simulink model "CM690A_HwAg0Meas"  (R2013b)
settings: Solver=FixedStepDiscrete  SolverMode=SingleTasking  StartTime=0.0  StopTime=22  FixedStep=0.002  RelTol=1e-3
undefined symbols (not defined in the file): ELECGLBPRM_DEGPERREV_DEGPERREV_F32, ELECGLBPRM_HWAGCENTROFFS_HWDEG_F32, ELECGLBPRM_HWAGSATNLOWRLIM_HWDEG_F32, ELECGLBPRM_HWAGSATNUPPRLIM_HWDEG_F32, ELECGLBPRM_HWAGSCA_ULS_F32, ELECGLBPRM_HWAGSPURGEARRAT_ULS_F32, ELECGLBPRM_HWAGSPURTORINGGEARRATSNSR0_ULS_F32, ELECGLBPRM_HWAGSPURTORINGGEARRATSNSR1_ULS_F32, ELECGLBPRM_NOFLT_CNT_U08, ELECGLBPRM_OFFSTRIMNOTPRFMD_CNT_U08, ELECGLBPRM_PRTCLFLT_CNT_U08, ELECGLBPRM_SKIPSTEPFLT_CNT_U08, ELECGLBPRM_SNSRINTFLT_CNT_U08, ELECGLBPRM_VRNRERRFLT_CNT_U08, FLTINJ_HWAG0MEAS_HWAG0, FLTINJ_HWAG0MEAS_TESTOK, HwAg0IfFlt, HwAg0MeasHwAg0IfFltFailStep, HwAg0MeasHwAg0IfFltPassStep, HwAg0MeasHwAg0Snsr0PrtclFltFailStep, HwAg0MeasHwAg0Snsr0PrtclFltPassStep, HwAg0MeasHwAg0Snsr1PrtclFltFailStep, HwAg0MeasHwAg0Snsr1PrtclFltPassStep, HwAg0MeasSnsr0Rev, HwAg0MeasSnsr1Rev, HwAg0MeasStep, HwAg0MeasVrnrErrThd, HwAg0MfgFlt, HwAg0Snsr0PrtclFlt, HwAg0Snsr1PrtclFlt, HWAG10THTOOTHTRIG_CNT_U08, HWAG11THTOOTHTRIG_CNT_U08, NtcSts1, sigbuilder_block, SigQlfr1
libraries: simulink x30, NxtrNvM x3
(part 4 of 5)

== system CM690A_HwAg0Meas/HwAg0Meas/HwAg0MeasPer2/Snsr0Read/RawHwAgRead/CopyRight2 ==

== system CM690A_HwAg0Meas/HwAg0Meas/HwAg0MeasPer2/Snsr0Read/RawHwAgRead/NewMsg ==
  note: Information Only:
      |
      | - Protocol Fault Evaluation
  note: ,
  note: Fault
      | Injection
      | Point
  Snsr0CS : Inport
  Snsr0FCCN : Inport  Port=2
  Snsr0Id : Inport  Port=3
  Snsr0Data : Inport  Port=4
  Action Port : ActionPort  ActionType=then
  Bus Creator : BusCreator  Inputs=3
  Bus Selector : BusSelector  OutputSignals=RawHwAg,TestOk,ParamByte
  Bus Selector1 : BusSelector  OutputSignals=RawHwAg,TestOk,ParamByte
  CopyRight2 : Subsystem  Description=|  mask(Copyright Information){none=on}
      | Copyright info block.                                               
      |                                                                     
      | Place copyright information at the top of every subsystem in design.
      mask prompts: none "No parameters"
      mask help: Place copyright information at the top of every subsystem in design.
      mask Display:
      | NxtrConf = 'Nexteer Confidential';
      | 
      | sys = bdroot; %handle for the current model ("system")
      | first = get_param(sys,'Created');
      | first = first(end-3:end);  %year is last four digits
      | 
      | last = get_param(sys,'LastModifiedDate');
      | if isempty(last)
      |     last = datestr(now,'yyyy');
      | else
      |     last = last(end-3:end);
      | end
      | 
      | if strcmp(first,last)
      |     fprintf('%s -- Copyright %s Nexteer',NxtrConf,first)
      | else
      |     fprintf('%s -- %s%s- %s Nexteer',NxtrConf,char(169),first,last)
      | end
  FIU : Constant  Value=FLTINJ_HWAG0MEAS_TESTOK
  FltInj_u08 : Subsystem  RequirementInfo={'linktype_rmi_doors' '0000cf45 (/ESG Group/FDD Module Requirements/EA4 Specific/CM690A_HwAg0Meas)' '#CM690A_109' 'true' 'REQ: CM690A_109' '' } %GIDa_7b346184_324c_480b_97a4_826e0f4ed5b6  TreatAsAtomicUnit=on  VariantControl=FltInj_sim  mask(Fault_Injection){}
      mask help: Fault Injection is a simulation only block for EA4 programs.
  If : If  RequirementInfo={} %GIDa_02db3ab5_be9b_4d14_aa60_e7f5bf325249  IfExpression=u1 == 0
  Merge : Merge
  Merge1 : Merge
  Merge2 : Merge
  NoStsFlt : Subsystem  RequirementInfo={} %GIDa_b7e9d759_3768_4543_969e_0ff60280fe32  TreatAsAtomicUnit=on
  STSFLT : Subsystem  RequirementInfo={'linktype_rmi_doors' '0000cf45 (/ESG Group/FDD Module Requirements/EA4 Specific/CM690A_HwAg0Meas)' '#CM690A_40' 'true' 'REQ: CM690A_40' '' ; 'linktype_rmi_doors' '0000cf45 (/ESG Group/FDD Module Requirements/EA4 Specific/CM690A_HwAg0Meas)' '#CM690A_41' 'true' 'REQ: CM690A_41' '' ; 'linktype_rmi_doors' '0000cf45 (/ESG Group/FDD Module Requirements/EA4 Specific/CM690A_HwAg0Meas)' '#CM690A_42' 'true' 'REQ: CM690A_42' '' ; 'linktype_rmi_doors' '0000cf45 (/ESG Group/FDD Module Requirements/EA4 Specific/CM690A_HwAg0Meas)' '#CM690A_43' 'true' 'REQ: CM690A_43' '' ; 'linktype_rmi_doors' '0000cf45 (/ESG Group/FDD Module Requirements/EA4 Specific/CM690A_HwAg0Meas)' '#CM690A_44' 'true' 'REQ: CM690A_44' '' ; 'linktype_rmi_doors' '0000cf45 (/ESG Group/FDD Module Requirements/EA4 Specific/CM690A_HwAg0Meas)' '#CM690A_89' 'true' 'REQ: CM690A_89' '' ; 'linktype_rmi_doors' '0000cf45 (/ESG Group/FDD Module Requirements/EA4 Specific/CM690A_HwAg0Meas)' '#CM690A_45' 'true' 'REQ: CM690A_45' '' ; 'linktype_rmi_doors' '0000cf45 (/ESG Group/FDD Module Requirements/EA4 Specific/CM690A_HwAg0Meas)' '#CM690A_46' 'true' 'REQ: CM690A_46' '' } %GIDa_15585e29_68a1_46d0_9954_0916d9066e3c  TreatAsAtomicUnit=on
      mask Display: disp('STSFLT')
  Out1 : Outport
  wires:
  Snsr0CS/1 -> FltInj_u08/1(Signal)
  If/1 -> NoStsFlt/Action  "NoFault"
  If/2 -> STSFLT/Action  "Fault"
  Merge/1 -> Bus Creator/2  "TestOk"
  Merge1/1 -> Bus Creator/3  "ParamByte"
  Merge2/1 -> Bus Creator/1  "RawHwAg"
  NoStsFlt/1(Out1) -> Bus Selector/1
  STSFLT/1(Out1) -> Bus Selector1/1
  Bus Selector1/1 -> Merge2/1  "<RawHwAg>"
  Bus Selector/1 -> Merge2/2  "<RawHwAg>"
  Bus Selector1/2 -> Merge/1  "<TestOk>"
  Bus Selector1/3 -> Merge1/1  "<ParamByte>"
  Bus Selector/2 -> Merge/2  "<TestOk>"
  Bus Selector/3 -> Merge1/2  "<ParamByte>"
  Bus Creator/1 -> Out1/1
  FIU/1 -> FltInj_u08/2(Const)
  FltInj_u08/1(Out1) -> If/1
  Snsr0FCCN/1 -> NoStsFlt/1(Snsr0FCCN)
  Snsr0Data/1 -> NoStsFlt/3(Snsr0Data)
  Snsr0Id/1 -> NoStsFlt/2(Snsr0Id)

== system CM690A_HwAg0Meas/HwAg0Meas/HwAg0MeasPer2/Snsr0Read/RawHwAgRead/NoNewMsg ==
  Action Port : ActionPort  ActionType=else
  Add : Sum
  Bus Creator : BusCreator  Inputs=3
  Constant : Constant  OutDataTypeStr=uint8
  CopyRight2 : Subsystem  Description=|  mask(Copyright Information){none=on}
      | Copyright info block.                                               
      |                                                                     
      | Place copyright information at the top of every subsystem in design.
      mask prompts: none "No parameters"
      mask help: Place copyright information at the top of every subsystem in design.
      mask Display:
      | NxtrConf = 'Nexteer Confidential';
      | 
      | sys = bdroot; %handle for the current model ("system")
      | first = get_param(sys,'Created');
      | first = first(end-3:end);  %year is last four digits
      | 
      | last = get_param(sys,'LastModifiedDate');
      | if isempty(last)
      |     last = datestr(now,'yyyy');
      | else
      |     last = last(end-3:end);
      | end
      | 
      | if strcmp(first,last)
      |     fprintf('%s -- Copyright %s Nexteer',NxtrConf,first)
      | else
      |     fprintf('%s -- %s%s- %s Nexteer',NxtrConf,char(169),first,last)
      | end
  Data Store Read : DataStoreRead  DataStoreName=HwAg0Snsr0NoMsgErrCntr
  Data Store Write : DataStoreWrite  DataStoreName=HwAg0Snsr0NoMsgErrCntr
  Data Type Conversion : DataTypeConversion  OutDataTypeStr=uint8
  HwAg : Constant  Value=0  OutDataTypeStr=uint16
  NtcSts : simulink/Sources/Enumerated Constant  OutDataTypeStr=Enum: NtcSts1  Value=NtcSts1.NTCSTS_PREFAILD  SampleTime=inf
  PRTCL_FAULT : Constant  Value=ELECGLBPRM_PRTCLFLT_CNT_U08  OutDataTypeStr=uint8
  Signal Conversion : SignalConversion
  Out1 : Outport
  wires:
  PRTCL_FAULT/1 -> Bus Creator/3  "ParamByte"
  NtcSts/1 -> Data Type Conversion/1
  HwAg/1 -> Bus Creator/1  "RawHwAg"
  Bus Creator/1 -> Signal Conversion/1
  Signal Conversion/1 -> Out1/1
  Data Type Conversion/1 -> Bus Creator/2  "TestOk"
  Data Store Read/1 -> Add/1
  Constant/1 -> Add/2
  Add/1 -> Data Store Write/1

== system CM690A_HwAg0Meas/HwAg0Meas/HwAg0MeasPer2/Snsr0Read/Read the Flag/CopyRight2 ==

== system CM690A_HwAg0Meas/HwAg0Meas/HwAg0MeasPer2/Snsr0Read/SetNtcSts/CopyRight2 ==

== system CM690A_HwAg0Meas/HwAg0Meas/HwAg0MeasPer3/Snsr1Read/DebStepSelection/CopyRight2 ==

== system CM690A_HwAg0Meas/HwAg0Meas/HwAg0MeasPer3/Snsr1Read/Do nothing1/CopyRight2 ==

== system CM690A_HwAg0Meas/HwAg0Meas/HwAg0MeasPer3/Snsr1Read/Do nothing2/CopyRight2 ==

== system CM690A_HwAg0Meas/HwAg0Meas/HwAg0MeasPer3/Snsr1Read/RawHwAgRead/CopyRight2 ==

== system CM690A_HwAg0Meas/HwAg0Meas/HwAg0MeasPer3/Snsr1Read/RawHwAgRead/NewMsg ==
  note: Information Only:
      |
      | - Protocol Fault Evaluation
  Snsr1CS : Inport
  Snsr1FCCN : Inport  Port=2
  Snsr1Id : Inport  Port=3
  Snsr1Data : Inport  Port=4
  Action Port : ActionPort  ActionType=then
  Bus Creator : BusCreator  Inputs=3
  Bus Selector : BusSelector  OutputSignals=RawHwAg,TestOk,ParamByte
  Bus Selector1 : BusSelector  OutputSignals=RawHwAg,TestOk,ParamByte
  CopyRight2 : Subsystem  Description=|  mask(Copyright Information){none=on}
      | Copyright info block.                                               
      |                                                                     
      | Place copyright information at the top of every subsystem in design.
      mask prompts: none "No parameters"
      mask help: Place copyright information at the top of every subsystem in design.
      mask Display:
      | NxtrConf = 'Nexteer Confidential';
      | 
      | sys = bdroot; %handle for the current model ("system")
      | first = get_param(sys,'Created');
      | first = first(end-3:end);  %year is last four digits
      | 
      | last = get_param(sys,'LastModifiedDate');
      | if isempty(last)
      |     last = datestr(now,'yyyy');
      | else
      |     last = last(end-3:end);
      | end
      | 
      | if strcmp(first,last)
      |     fprintf('%s -- Copyright %s Nexteer',NxtrConf,first)
      | else
      |     fprintf('%s -- %s%s- %s Nexteer',NxtrConf,char(169),first,last)
      | end
  If : If  RequirementInfo={} %GIDa_d01d7976_4a86_48f6_8a8d_571e55869e77  IfExpression=u1 == 0
  Merge : Merge
  Merge1 : Merge
  Merge2 : Merge
  NoStsFlt : Subsystem  RequirementInfo={} %GIDa_74b744eb_a548_4ce6_ac8b_09cb9d78172d  TreatAsAtomicUnit=on
  STSFLT : Subsystem  RequirementInfo={'linktype_rmi_doors' '0000cf45 (/ESG Group/FDD Module Requirements/EA4 Specific/CM690A_HwAg0Meas)' '#CM690A_57' 'true' 'REQ: CM690A_57' '' ; 'linktype_rmi_doors' '0000cf45 (/ESG Group/FDD Module Requirements/EA4 Specific/CM690A_HwAg0Meas)' '#CM690A_58' 'true' 'REQ: CM690A_58' '' ; 'linktype_rmi_doors' '0000cf45 (/ESG Group/FDD Module Requirements/EA4 Specific/CM690A_HwAg0Meas)' '#CM690A_59' 'true' 'REQ: CM690A_59' '' ; 'linktype_rmi_doors' '0000cf45 (/ESG Group/FDD Module Requirements/EA4 Specific/CM690A_HwAg0Meas)' '#CM690A_60' 'true' 'REQ: CM690A_60' '' ; 'linktype_rmi_doors' '0000cf45 (/ESG Group/FDD Module Requirements/EA4 Specific/CM690A_HwAg0Meas)' '#CM690A_61' 'true' 'REQ: CM690A_61' '' ; 'linktype_rmi_doors' '0000cf45 (/ESG Group/FDD Module Requirements/EA4 Specific/CM690A_HwAg0Meas)' '#CM690A_88' 'true' 'REQ: CM690A_88' '' ; 'linktype_rmi_doors' '0000cf45 (/ESG Group/FDD Module Requirements/EA4 Specific/CM690A_HwAg0Meas)' '#CM690A_62' 'true' 'REQ: CM690A_62' '' ; 'linktype_rmi_doors' '0000cf45 (/ESG Group/FDD Module Requirements/EA4 Specific/CM690A_HwAg0Meas)' '#CM690A_63' 'true' 'REQ: CM690A_63' '' } %GIDa_c06f9169_73b8_4668_a7a1_c8699a32a709  TreatAsAtomicUnit=on
      mask Display: disp('STSFLT')
  Out1 : Outport
  wires:
  If/1 -> NoStsFlt/Action  "NoFault"
  If/2 -> STSFLT/Action  "Fault"
  Merge/1 -> Bus Creator/2  "TestOk"
  Merge1/1 -> Bus Creator/3  "ParamByte"
  Merge2/1 -> Bus Creator/1  "RawHwAg"
  NoStsFlt/1(Out1) -> Bus Selector/1
  STSFLT/1(Out1) -> Bus Selector1/1
  Bus Selector1/1 -> Merge2/1  "<RawHwAg>"
  Bus Selector/1 -> Merge2/2  "<RawHwAg>"
  Bus Selector1/2 -> Merge/1  "<TestOk>"
  Bus Selector1/3 -> Merge1/1  "<ParamByte>"
  Bus Selector/2 -> Merge/2  "<TestOk>"
  Bus Selector/3 -> Merge1/2  "<ParamByte>"
  Bus Creator/1 -> Out1/1
  Snsr1CS/1 -> If/1
  Snsr1FCCN/1 -> NoStsFlt/1(Snsr1FCCN)
  Snsr1Data/1 -> NoStsFlt/3(Snsr1Data)
  Snsr1Id/1 -> NoStsFlt/2(Snsr1Id)

== stateflow chart CM690A_HwAg0Meas/HwAg0Meas/HwAg0MeasPer4/HwAgRead/HwAg0Final/ModRoll ==
  settings: stateMachineType=MEALY_MACHINE
  note: Nexteer Automotive Confidential
  (default) -> (junction 89)
  (junction 89) -> (junction 93) [order 2] : [ RawVal>900 ]
      | {OutVal = RawVal-1800;}
  (junction 89) -> (junction 93) [order 3] : {OutVal = RawVal;}
  (junction 89) -> (junction 93) [order 1] : [RawVal<-900 ]
      | {OutVal = RawVal+1800;}
  data: OutVal output single; RawVal input single

== system CM690A_HwAg0Meas/HwAg0Meas/HwAg0MeasPer3/Snsr1Read/RawHwAgRead/NoNewMsg ==
  Action Port : ActionPort  ActionType=else
  Add : Sum
  Bus Creator : BusCreator  Inputs=3
  Constant : Constant  OutDataTypeStr=uint8
  CopyRight2 : Subsystem  Description=|  mask(Copyright Information){none=on}
      | Copyright info block.                                               
      |                                                                     
      | Place copyright information at the top of every subsystem in design.
      mask prompts: none "No parameters"
      mask help: Place copyright information at the top of every subsystem in design.
      mask Display:
      | NxtrConf = 'Nexteer Confidential';
      | 
      | sys = bdroot; %handle for the current model ("system")
      | first = get_param(sys,'Created');
      | first = first(end-3:end);  %year is last four digits
      | 
      | last = get_param(sys,'LastModifiedDate');
      | if isempty(last)
      |     last = datestr(now,'yyyy');
      | else
      |     last = last(end-3:end);
      | end
      | 
      | if strcmp(first,last)
      |     fprintf('%s -- Copyright %s Nexteer',NxtrConf,first)
      | else
      |     fprintf('%s -- %s%s- %s Nexteer',NxtrConf,char(169),first,last)
      | end
  Data Store Read : DataStoreRead  DataStoreName=HwAg0Snsr1NoMsgErrCntr
  Data Store Write : DataStoreWrite  DataStoreName=HwAg0Snsr1NoMsgErrCntr
  Data Type Conversion : DataTypeConversion  OutDataTypeStr=uint8
  HwAg : Constant  Value=0  OutDataTypeStr=uint16
  NtcSts : simulink/Sources/Enumerated Constant  OutDataTypeStr=Enum: NtcSts1  Value=NtcSts1.NTCSTS_PREFAILD  SampleTime=inf
  PRTCL_FAULT : Constant  Value=ELECGLBPRM_PRTCLFLT_CNT_U08  OutDataTypeStr=uint8
  Signal Conversion : SignalConversion
  Out1 : Outport
  wires:
  PRTCL_FAULT/1 -> Bus Creator/3  "ParamByte"
  NtcSts/1 -> Data Type Conversion/1
  HwAg/1 -> Bus Creator/1  "RawHwAg"
  Bus Creator/1 -> Signal Conversion/1
  Signal Conversion/1 -> Out1/1
  Data Type Conversion/1 -> Bus Creator/2  "TestOk"
  Data Store Read/1 -> Add/1
  Constant/1 -> Add/2
  Add/1 -> Data Store Write/1

== system CM690A_HwAg0Meas/HwAg0Meas/HwAg0MeasPer3/Snsr1Read/Read the Flag/CopyRight2 ==

== system CM690A_HwAg0Meas/HwAg0Meas/HwAg0MeasPer3/Snsr1Read/SetNtcSts/CopyRight2 ==

== system CM690A_HwAg0Meas/HwAg0Meas/HwAg0MeasPer3/Snsr1Read/SyncPulse/CopyRight2 ==

== system CM690A_HwAg0Meas/HwAg0Meas/HwAg0MeasPer3/Snsr1Read/SyncPulse/GetRefTmr1MicroSec32bit ==
  CopyRight2 : Subsystem  Description=|  mask(Copyright Information){none=on}
      | Copyright info block.                                               
      |                                                                     
      | Place copyright information at the top of every subsystem in design.
      mask prompts: none "No parameters"
      mask help: Place copyright information at the top of every subsystem in design.
      mask Display:
      | NxtrConf = 'Nexteer Confidential';
      | 
      | sys = bdroot; %handle for the current model ("system")
      | first = get_param(sys,'Created');
      | first = first(end-3:end);  %year is last four digits
      | 
      | last = get_param(sys,'LastModifiedDate');
      | if isempty(last)
      |     last = datestr(now,'yyyy');
      | else
      |     last = last(end-3:end);
      | end
      | 
      | if strcmp(first,last)
      |     fprintf('%s -- Copyright %s Nexteer',NxtrConf,first)
      | else
      |     fprintf('%s -- %s%s- %s Nexteer',NxtrConf,char(169),first,last)
      | end
  Ground : Ground
  RefTmr : Outport
  wires:
  Ground/1 -> RefTmr/1

== system CM690A_HwAg0Meas/HwAg0Meas/HwAg0MeasPer3/Snsr1Read/SyncPulse/GetTiSpan1MicroSec32bit ==
  RefTmr : Inport
  CopyRight2 : Subsystem  Description=|  mask(Copyright Information){none=on}
      | Copyright info block.                                               
      |                                                                     
      | Place copyright information at the top of every subsystem in design.
      mask prompts: none "No parameters"
      mask help: Place copyright information at the top of every subsystem in design.
      mask Display:
      | NxtrConf = 'Nexteer Confidential';
      | 
      | sys = bdroot; %handle for the current model ("system")
      | first = get_param(sys,'Created');
      | first = first(end-3:end);  %year is last four digits
      | 
      | last = get_param(sys,'LastModifiedDate');
      | if isempty(last)
      |     last = datestr(now,'yyyy');
      | else
      |     last = last(end-3:end);
      | end
      | 
      | if strcmp(first,last)
      |     fprintf('%s -- Copyright %s Nexteer',NxtrConf,first)
      | else
      |     fprintf('%s -- %s%s- %s Nexteer',NxtrConf,char(169),first,last)
      | end
  Ground : Ground
  Terminator : Terminator
  TiSpan : Outport
  wires:
  RefTmr/1 -> Terminator/1
  Ground/1 -> TiSpan/1

== system CM690A_HwAg0Meas/HwAg0Meas/HwAg0MeasPer4/HwAgRead/GetNtcQlfr/CopyRight2 ==

== system CM690A_HwAg0Meas/HwAg0Meas/HwAg0MeasPer4/HwAgRead/GetNtcQlfr1/CopyRight2 ==

== system CM690A_HwAg0Meas/HwAg0Meas/HwAg0MeasPer4/HwAgRead/GetNtcQlfr2/CopyRight2 ==

== system CM690A_HwAg0Meas/HwAg0Meas/HwAg0MeasPer4/HwAgRead/GetNtcQlfr3/CopyRight2 ==

== system CM690A_HwAg0Meas/HwAg0Meas/HwAg0MeasPer4/HwAgRead/HwAg0Final/CopyRight2 ==

== system CM690A_HwAg0Meas/HwAg0Meas/HwAg0MeasPer4/HwAgRead/If Action Subsystem/AdjStepCalc ==
  HwAg0Snsr0Rel : Inport
  HwAg0Sns1Rel : Inport  Port=2
  CopyRight2 : Subsystem  Description=|  mask(Copyright Information){none=on}
      | Copyright info block.                                               
      |                                                                     
      | Place copyright information at the top of every subsystem in design.
      mask prompts: none "No parameters"
      mask help: Place copyright information at the top of every subsystem in design.
      mask Display:
      | NxtrConf = 'Nexteer Confidential';
      | 
      | sys = bdroot; %handle for the current model ("system")
      | first = get_param(sys,'Created');
      | first = first(end-3:end);  %year is last four digits
      | 
      | last = get_param(sys,'LastModifiedDate');
      | if isempty(last)
      |     last = datestr(now,'yyyy');
      | else
      |     last = last(end-3:end);
      | end
      | 
      | if strcmp(first,last)
      |     fprintf('%s -- Copyright %s Nexteer',NxtrConf,first)
      | else
      |     fprintf('%s -- %s%s- %s Nexteer',NxtrConf,char(169),first,last)
      | end
  Diagc : Subsystem
  InitStep : Subsystem
      settings: AttributesFormatString=%<Description>
  Intpn : Subsystem
  HwAg0 : Outport  OutDataTypeStr=single
  TestOk : Outport  Port=2  OutDataTypeStr=uint8
  ParamByte : Outport  Port=3
  wires:
  HwAg0Sns1Rel/1 -> Diagc/2(HwAg0Snsr1Rel), Intpn/2(HwAg0Snsr1Rel)
  HwAg0Snsr0Rel/1 -> Intpn/1(HwAg0Snsr0Rel), Diagc/1(HwAg0Snsr0Rel)
  Diagc/1(HwAg0) -> HwAg0/1
  Diagc/2(TestOk) -> TestOk/1
  Diagc/3(ParamByte) -> ParamByte/1
  Intpn/1(HwAg0Snsr0Rev) -> Diagc/3(HwAg0Snsr0Rev)
  Intpn/2(HwAg0Snsr1Rev) -> Diagc/4(HwAg0Snsr1Rev)
  Intpn/3(HwAg0StepSeqNr) -> InitStep/1(HwAg0StepSeqNr_In)
  InitStep/1(HwAg0StepSeqNr_Out) -> Diagc/5(HwAg0StepSeqNr)

== system CM690A_HwAg0Meas/HwAg0Meas/HwAg0MeasPer4/HwAgRead/If Action Subsystem/CopyRight2 ==

== system CM690A_HwAg0Meas/HwAg0Meas/HwAg0MeasPer4/HwAgRead/If Action Subsystem/DebStepSelection ==
  TestOk : Inport
  CopyRight2 : Subsystem  Description=|  mask(Copyright Information){none=on}
      | Copyright info block.                                               
      |                                                                     
      | Place copyright information at the top of every subsystem in design.
      mask prompts: none "No parameters"
      mask help: Place copyright information at the top of every subsystem in design.
      mask Display:
      | NxtrConf = 'Nexteer Confidential';
      | 
      | sys = bdroot; %handle for the current model ("system")
      | first = get_param(sys,'Created');
      | first = first(end-3:end);  %year is last four digits
      | 
      | last = get_param(sys,'LastModifiedDate');
      | if isempty(last)
      |     last = datestr(now,'yyyy');
      | else
      |     last = last(end-3:end);
      | end
      | 
      | if strcmp(first,last)
      |     fprintf('%s -- Copyright %s Nexteer',NxtrConf,first)
      | else
      |     fprintf('%s -- %s%s- %s Nexteer',NxtrConf,char(169),first,last)
      | end
  NTCFailStepCal : Constant  Value=HwAg0MeasHwAg0IfFltFailStep
  NTCPassStepCal : Constant  Value=HwAg0MeasHwAg0IfFltPassStep
  Switch : Switch  Criteria=u2 > Threshold  Threshold=2
  DebStep : Outport  OutDataTypeStr=uint16
  wires:
  NTCFailStepCal/1 -> Switch/1
  Switch/1 -> DebStep/1
  NTCPassStepCal/1 -> Switch/3
  TestOk/1 -> Switch/2

== system CM690A_HwAg0Meas/HwAg0Meas/HwAg0MeasPer4/HwAgRead/If Action Subsystem/HwAg0Snsr0RelCalc ==
  RawHwAg0Snsr0 : Inport
  CopyRight2 : Subsystem  Description=|  mask(Copyright Information){none=on}
      | Copyright info block.                                               
      |                                                                     
      | Place copyright information at the top of every subsystem in design.
      mask prompts: none "No parameters"
      mask help: Place copyright information at the top of every subsystem in design.
      mask Display:
      | NxtrConf = 'Nexteer Confidential';
      | 
      | sys = bdroot; %handle for the current model ("system")
      | first = get_param(sys,'Created');
      | first = first(end-3:end);  %year is last four digits
      | 
      | last = get_param(sys,'LastModifiedDate');
      | if isempty(last)
      |     last = datestr(now,'yyyy');
      | else
      |     last = last(end-3:end);
      | end
      | 
      | if strcmp(first,last)
      |     fprintf('%s -- Copyright %s Nexteer',NxtrConf,first)
      | else
      |     fprintf('%s -- %s%s- %s Nexteer',NxtrConf,char(169),first,last)
      | end
  Data Type Conversion1 : DataTypeConversion  OutDataTypeStr=single
  HwAgSca : Constant  Value=ELECGLBPRM_HWAGSCA_ULS_F32  OutDataTypeStr=single
  PIM : DataStoreWrite  RequirementInfo={'linktype_rmi_doors' '0000cf45 (/ESG Group/FDD Module Requirements/EA4 Specific/CM690A_HwAg0Meas)' '#CM690A_91' 'true' 'REQ: CM690A_91' '' } %GIDa_59d01f39_63a3_4259_af30_74d2175aa8e2  DataStoreName=dHwAg0MeasSnsr0Rel
  Product : Product
  HwAg0Snsr0Rel : Outport  OutDataTypeStr=single
  wires:
  Data Type Conversion1/1 -> Product/1
  RawHwAg0Snsr0/1 -> Data Type Conversion1/1
  HwAgSca/1 -> Product/2
  Product/1 -> PIM/1, HwAg0Snsr0Rel/1

== system CM690A_HwAg0Meas/HwAg0Meas/HwAg0MeasPer4/HwAgRead/If Action Subsystem/HwAg0Snsr1RelCalc ==
  RawHwAg0Snsr1 : Inport
  CopyRight2 : Subsystem  Description=|  mask(Copyright Information){none=on}
      | Copyright info block.                                               
      |                                                                     
      | Place copyright information at the top of every subsystem in design.
      mask prompts: none "No parameters"
      mask help: Place copyright information at the top of every subsystem in design.
      mask Display:
      | NxtrConf = 'Nexteer Confidential';
      | 
      | sys = bdroot; %handle for the current model ("system")
      | first = get_param(sys,'Created');
      | first = first(end-3:end);  %year is last four digits
      | 
      | last = get_param(sys,'LastModifiedDate');
      | if isempty(last)
      |     last = datestr(now,'yyyy');
      | else
      |     last = last(end-3:end);
      | end
      | 
      | if strcmp(first,last)
      |     fprintf('%s -- Copyright %s Nexteer',NxtrConf,first)
      | else
      |     fprintf('%s -- %s%s- %s Nexteer',NxtrConf,char(169),first,last)
      | end
  Data Type Conversion1 : DataTypeConversion  OutDataTypeStr=single
  HwAgSca : Constant  Value=ELECGLBPRM_HWAGSCA_ULS_F32  OutDataTypeStr=single
  PIM : DataStoreWrite  RequirementInfo={'linktype_rmi_doors' '0000cf45 (/ESG Group/FDD Module Requirements/EA4 Specific/CM690A_HwAg0Meas)' '#CM690A_91' 'true' 'REQ: CM690A_91' '' } %GIDa_1b631432_d95a_4a43_9f9d_f4fe0e6172af  DataStoreName=dHwAg0MeasSnsr1Rel
  Product : Product
  HwAg0Snsr1Rel : Outport  OutDataTypeStr=single
  wires:
  Data Type Conversion1/1 -> Product/1
  RawHwAg0Snsr1/1 -> Data Type Conversion1/1
  HwAgSca/1 -> Product/2
  Product/1 -> PIM/1, HwAg0Snsr1Rel/1

== system CM690A_HwAg0Meas/HwAg0Meas/HwAg0MeasPer4/HwAgRead/If Action Subsystem/SetNtcSts ==
  note: Note:
      |
      | - "ISO Fault Debounce Design" Simulink block intent to use here for Simulation purpose only. Do not Code this block
  NtcNr : Inport
  NtcStInfo : Inport  Port=2
  NtcSts : Inport  Port=3
  DebStep : Inport  Port=4
  CopyRight2 : Subsystem  Description=|  mask(Copyright Information){none=on}
      | Copyright info block.                                               
      |                                                                     
      | Place copyright information at the top of every subsystem in design.
      mask prompts: none "No parameters"
      mask help: Place copyright information at the top of every subsystem in design.
      mask Display:
      | NxtrConf = 'Nexteer Confidential';
      | 
      | sys = bdroot; %handle for the current model ("system")
      | first = get_param(sys,'Created');
      | first = first(end-3:end);  %year is last four digits
      | 
      | last = get_param(sys,'LastModifiedDate');
      | if isempty(last)
      |     last = datestr(now,'yyyy');
      | else
      |     last = last(end-3:end);
      | end
      | 
      | if strcmp(first,last)
      |     fprintf('%s -- Copyright %s Nexteer',NxtrConf,first)
      | else
      |     fprintf('%s -- %s%s- %s Nexteer',NxtrConf,char(169),first,last)
      | end
  Data Store Write : DataStoreWrite  DataStoreName=Ntc0x094Qlfr
  Ground : Ground
  ISO Fault Debounce Design : Stateflow chart  TreatAsAtomicUnit=on
      settings: AttributesFormatString=|
      | Simulation Purpose Only.
      | Do Not Code this block
      | Diagnostic Manager Owns this requirement
  Scope1 : Scope  NumInputPorts=3
      settings: YMin=-5~-5~-5  YMax=5~5~5  SaveName=ScopeData5
  Terminator : Terminator
  Terminator1 : Terminator
  wires:
  Ground/1 -> ISO Fault Debounce Design/3(SvcClr)
  ISO Fault Debounce Design/1(Qualifier) -> Data Store Write/1, Scope1/3
  DebStep/1 -> Scope1/2, ISO Fault Debounce Design/2(DebStep)
  NtcSts/1 -> Scope1/1, ISO Fault Debounce Design/1(NtcSts)
  NtcNr/1 -> Terminator/1
  NtcStInfo/1 -> Terminator1/1

== system CM690A_HwAg0Meas/HwAg0Meas/HwAg0MeasPer4/HwAgRead/If Action Subsystem1/CopyRight2 ==

== system CM690A_HwAg0Meas/HwAg0Meas/HwAg0MeasPer4/HwAgRead/If Action Subsystem2/CopyRight2 ==

== system CM690A_HwAg0Meas/HwAg0Meas/HwAg0MeasPer4/HwAgRead/If Action Subsystem3/CopyRight2 ==

== system CM690A_HwAg0Meas/HwAg0Meas/HwAg0MeasPer2/Snsr0Read/RawHwAgRead/NewMsg/CopyRight2 ==

== system CM690A_HwAg0Meas/HwAg0Meas/HwAg0MeasPer2/Snsr0Read/RawHwAgRead/NewMsg/FltInj_u08 ==
  note: Inport #2 must be constant
      | Const: FltInjectionLocType
  note: EA4.x Fault Injection
  note: This block requires no modification by FDD author.
      |
      | This block does not actually simulate any fault injection.  It is simply a pass-thru.
      |
      | The Const port (#2) simply terminates its signal, but we are trying to force the FDD author
      | to properly use the FltInjectionLocType enumeration in FDD model.
  Signal : Inport
  Const : Inport  Port=2
  Terminator : Terminator
  Out1 : Outport
  wires:
  Const/1 -> Terminator/1
  Signal/1 -> Out1/1

== system CM690A_HwAg0Meas/HwAg0Meas/HwAg0MeasPer2/Snsr0Read/RawHwAgRead/NewMsg/NoStsFlt ==
  note: Information Only:
      |
      | - Sensor Internal Fault (Status and Communication Nibble)
  Snsr0FCCN : Inport
  Snsr0Id : Inport  Port=2
  Snsr0Data : Inport  Port=3
  Action Port : ActionPort  ActionType=then
  Bus Creator : BusCreator  Inputs=3
  Bus Selector : BusSelector  OutputSignals=RawHwAg,TestOk,ParamByte
  Bus Selector1 : BusSelector  OutputSignals=RawHwAg,TestOk,ParamByte
  CommFlt : Subsystem  RequirementInfo={'linktype_rmi_doors' '0000cf45 (/ESG Group/FDD Module Requirements/EA4 Specific/CM690A_HwAg0Meas)' '#CM690A_28' 'true' 'REQ: CM690A_28' '' ; 'linktype_rmi_doors' '0000cf45 (/ESG Group/FDD Module Requirements/EA4 Specific/CM690A_HwAg0Meas)' '#CM690A_48' 'true' 'REQ: CM690A_48' '' } %GIDa_aa2d37a4_ae50_4823_85d7_2cd44654be8c  TreatAsAtomicUnit=on
      mask Display: disp('CommFlt')
  CopyRight2 : Subsystem  Description=|  mask(Copyright Information){none=on}
      | Copyright info block.                                               
      |                                                                     
      | Place copyright information at the top of every subsystem in design.
      mask prompts: none "No parameters"
      mask help: Place copyright information at the top of every subsystem in design.
      mask Display:
      | NxtrConf = 'Nexteer Confidential';
      | 
      | sys = bdroot; %handle for the current model ("system")
      | first = get_param(sys,'Created');
      | first = first(end-3:end);  %year is last four digits
      | 
      | last = get_param(sys,'LastModifiedDate');
      | if isempty(last)
      |     last = datestr(now,'yyyy');
      | else
      |     last = last(end-3:end);
      | end
      | 
      | if strcmp(first,last)
      |     fprintf('%s -- Copyright %s Nexteer',NxtrConf,first)
      | else
      |     fprintf('%s -- %s%s- %s Nexteer',NxtrConf,char(169),first,last)
      | end
  If : If  IfExpression=u1 == 0
  Merge : Merge
  Merge1 : Merge
  Merge2 : Merge
  TestPass : Subsystem  TreatAsAtomicUnit=on
  Out1 : Outport
  wires:
  Snsr0FCCN/1 -> If/1
  If/1 -> TestPass/Action
  If/2 -> CommFlt/Action
  Merge/1 -> Bus Creator/2  "TestOk"
  Merge1/1 -> Bus Creator/3  "ParamByte"
  Merge2/1 -> Bus Creator/1  "RawHwAg"
  TestPass/1(Out1) -> Bus Selector/1
  CommFlt/1(Out2) -> Bus Selector1/1
  Bus Selector1/1 -> Merge2/1  "<RawHwAg>"
  Bus Selector/1 -> Merge2/2  "<RawHwAg>"
  Bus Selector1/2 -> Merge/1  "<TestOk>"
  Bus Selector1/3 -> Merge1/1  "<ParamByte>"
  Bus Selector/2 -> Merge/2  "<TestOk>"
  Bus Selector/3 -> Merge1/2  "<ParamByte>"
  Bus Creator/1 -> Out1/1
  Snsr0Data/1 -> TestPass/2(Snsr0Data)
  Snsr0Id/1 -> TestPass/1(Snsr0Id)

== system CM690A_HwAg0Meas/HwAg0Meas/HwAg0MeasPer2/Snsr0Read/RawHwAgRead/NewMsg/STSFLT ==
  Action Port : ActionPort  ActionType=else
  Add : Sum
  Bus Creator : BusCreator  Inputs=3
  Constant : Constant  OutDataTypeStr=uint8
  CopyRight2 : Subsystem  Description=|  mask(Copyright Information){none=on}
      | Copyright info block.                                               
      |                                                                     
      | Place copyright information at the top of every subsystem in design.
      mask prompts: none "No parameters"
      mask help: Place copyright information at the top of every subsystem in design.
      mask Display:
      | NxtrConf = 'Nexteer Confidential';
      | 
      | sys = bdroot; %handle for the current model ("system")
      | first = get_param(sys,'Created');
      | first = first(end-3:end);  %year is last four digits
      | 
      | last = get_param(sys,'LastModifiedDate');
      | if isempty(last)
      |     last = datestr(now,'yyyy');
      | else
      |     last = last(end-3:end);
      | end
      | 
      | if strcmp(first,last)
      |     fprintf('%s -- Copyright %s Nexteer',NxtrConf,first)
      | else
      |     fprintf('%s -- %s%s- %s Nexteer',NxtrConf,char(169),first,last)
      | end
  Data Store Read : DataStoreRead  DataStoreName=HwAg0Snsr0ComStsErrCntr
  Data Store Write : DataStoreWrite  DataStoreName=HwAg0Snsr0ComStsErrCntr
  Data Type Conversion : DataTypeConversion  OutDataTypeStr=uint8
  HwAg : Constant  Value=0  OutDataTypeStr=uint16
  NtcSts : simulink/Sources/Enumerated Constant  OutDataTypeStr=Enum: NtcSts1  Value=NtcSts1.NTCSTS_PREFAILD  SampleTime=inf
  PRTCL_FAULT : Constant  Value=ELECGLBPRM_PRTCLFLT_CNT_U08  OutDataTypeStr=uint8
  Signal Conversion : SignalConversion
  Out1 : Outport
  wires:
  PRTCL_FAULT/1 -> Bus Creator/3  "ParamByte"
  NtcSts/1 -> Data Type Conversion/1
  HwAg/1 -> Bus Creator/1  "RawHwAg"
  Bus Creator/1 -> Signal Conversion/1
  Signal Conversion/1 -> Out1/1
  Data Type Conversion/1 -> Bus Creator/2  "TestOk"
  Data Store Read/1 -> Add/1
  Constant/1 -> Add/2
  Add/1 -> Data Store Write/1

== system CM690A_HwAg0Meas/HwAg0Meas/HwAg0MeasPer2/Snsr0Read/RawHwAgRead/NoNewMsg/CopyRight2 ==

== system CM690A_HwAg0Meas/HwAg0Meas/HwAg0MeasPer3/Snsr1Read/RawHwAgRead/NewMsg/CopyRight2 ==

== system CM690A_HwAg0Meas/HwAg0Meas/HwAg0MeasPer3/Snsr1Read/RawHwAgRead/NewMsg/NoStsFlt ==
  note: Information Only:
      |
      | - Sensor Internal Fault (Status and Communication Nibble)
  Snsr1FCCN : Inport
  Snsr1Id : Inport  Port=2
  Snsr1Data : Inport  Port=3
  Action Port : ActionPort  ActionType=then
  Bus Creator : BusCreator  Inputs=3
  Bus Selector : BusSelector  OutputSignals=RawHwAg,TestOk,ParamByte
  Bus Selector1 : BusSelector  OutputSignals=RawHwAg,TestOk,ParamByte
  CommFlt : Subsystem  RequirementInfo={'linktype_rmi_doors' '0000cf45 (/ESG Group/FDD Module Requirements/EA4 Specific/CM690A_HwAg0Meas)' '#CM690A_65' 'true' 'REQ: CM690A_65' '' } %GIDa_4aa8a7c8_592a_4e61_9fe7_e51e9f599cc1  TreatAsAtomicUnit=on
      mask Display: disp('CommFlt')
  CopyRight2 : Subsystem  Description=|  mask(Copyright Information){none=on}
      | Copyright info block.                                               
      |                                                                     
      | Place copyright information at the top of every subsystem in design.
      mask prompts: none "No parameters"
      mask help: Place copyright information at the top of every subsystem in design.
      mask Display:
      | NxtrConf = 'Nexteer Confidential';
      | 
      | sys = bdroot; %handle for the current model ("system")
      | first = get_param(sys,'Created');
      | first = first(end-3:end);  %year is last four digits
      | 
      | last = get_param(sys,'LastModifiedDate');
      | if isempty(last)
      |     last = datestr(now,'yyyy');
      | else
      |     last = last(end-3:end);
      | end
      | 
      | if strcmp(first,last)
      |     fprintf('%s -- Copyright %s Nexteer',NxtrConf,first)
      | else
      |     fprintf('%s -- %s%s- %s Nexteer',NxtrConf,char(169),first,last)
      | end
  If : If  IfExpression=u1 == 0
  Merge : Merge
  Merge1 : Merge
  Merge2 : Merge
  TestPass : Subsystem  TreatAsAtomicUnit=on
  Out1 : Outport
  wires:
  Snsr1FCCN/1 -> If/1
  If/1 -> TestPass/Action
  If/2 -> CommFlt/Action
  Merge/1 -> Bus Creator/2  "TestOk"
  Merge1/1 -> Bus Creator/3  "ParamByte"
  Merge2/1 -> Bus Creator/1  "RawHwAg"
  TestPass/1(Out1) -> Bus Selector/1
  CommFlt/1(Out2) -> Bus Selector1/1
  Bus Selector1/1 -> Merge2/1  "<RawHwAg>"
  Bus Selector/1 -> Merge2/2  "<RawHwAg>"
  Bus Selector1/2 -> Merge/1  "<TestOk>"
  Bus Selector1/3 -> Merge1/1  "<ParamByte>"
  Bus Selector/2 -> Merge/2  "<TestOk>"
  Bus Selector/3 -> Merge1/2  "<ParamByte>"
  Bus Creator/1 -> Out1/1
  Snsr1Data/1 -> TestPass/2(Snsr1Data)
  Snsr1Id/1 -> TestPass/1(Snsr1Id)

== system CM690A_HwAg0Meas/HwAg0Meas/HwAg0MeasPer3/Snsr1Read/RawHwAgRead/NewMsg/STSFLT ==
  Action Port : ActionPort  ActionType=else
  Add : Sum
  Bus Creator : BusCreator  Inputs=3
  Constant : Constant  OutDataTypeStr=uint8
  CopyRight2 : Subsystem  Description=|  mask(Copyright Information){none=on}
      | Copyright info block.                                               
      |                                                                     
      | Place copyright information at the top of every subsystem in design.
      mask prompts: none "No parameters"
      mask help: Place copyright information at the top of every subsystem in design.
      mask Display:
      | NxtrConf = 'Nexteer Confidential';
      | 
      | sys = bdroot; %handle for the current model ("system")
      | first = get_param(sys,'Created');
      | first = first(end-3:end);  %year is last four digits
      | 
      | last = get_param(sys,'LastModifiedDate');
      | if isempty(last)
      |     last = datestr(now,'yyyy');
      | else
      |     last = last(end-3:end);
      | end
      | 
      | if strcmp(first,last)
      |     fprintf('%s -- Copyright %s Nexteer',NxtrConf,first)
      | else
      |     fprintf('%s -- %s%s- %s Nexteer',NxtrConf,char(169),first,last)
      | end
  Data Store Read : DataStoreRead  DataStoreName=HwAg0Snsr1ComStsErrCntr
  Data Store Write : DataStoreWrite  DataStoreName=HwAg0Snsr1ComStsErrCntr
  Data Type Conversion : DataTypeConversion  OutDataTypeStr=uint8
  HwAg : Constant  Value=0  OutDataTypeStr=uint16
  NtcSts : simulink/Sources/Enumerated Constant  OutDataTypeStr=Enum: NtcSts1  Value=NtcSts1.NTCSTS_PREFAILD  SampleTime=inf
  PRTCL_FAULT : Constant  Value=ELECGLBPRM_PRTCLFLT_CNT_U08  OutDataTypeStr=uint8
  Signal Conversion : SignalConversion
  Out1 : Outport
  wires:
  PRTCL_FAULT/1 -> Bus Creator/3  "ParamByte"
  NtcSts/1 -> Data Type Conversion/1
  HwAg/1 -> Bus Creator/1  "RawHwAg"
  Bus Creator/1 -> Signal Conversion/1
  Signal Conversion/1 -> Out1/1
  Data Type Conversion/1 -> Bus Creator/2  "TestOk"
  Data Store Read/1 -> Add/1
  Constant/1 -> Add/2
  Add/1 -> Data Store Write/1

== system CM690A_HwAg0Meas/HwAg0Meas/HwAg0MeasPer3/Snsr1Read/RawHwAgRead/NoNewMsg/CopyRight2 ==

== system CM690A_HwAg0Meas/HwAg0Meas/HwAg0MeasPer3/Snsr1Read/SyncPulse/GetRefTmr1MicroSec32bit/CopyRight2 ==

== system CM690A_HwAg0Meas/HwAg0Meas/HwAg0MeasPer3/Snsr1Read/SyncPulse/GetTiSpan1MicroSec32bit/CopyRight2 ==

== system CM690A_HwAg0Meas/HwAg0Meas/HwAg0MeasPer4/HwAgRead/If Action Subsystem/AdjStepCalc/CopyRight2 ==

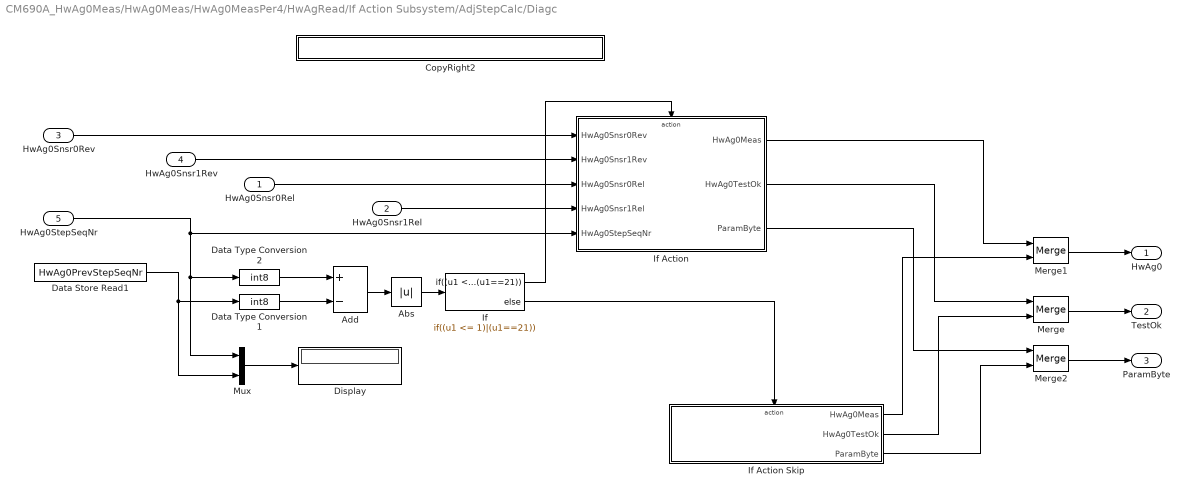
== system CM690A_HwAg0Meas/HwAg0Meas/HwAg0MeasPer4/HwAgRead/If Action Subsystem/AdjStepCalc/Diagc ==
  HwAg0Snsr0Rel : Inport
  HwAg0Snsr1Rel : Inport  Port=2
  HwAg0Snsr0Rev : Inport  Port=3
  HwAg0Snsr1Rev : Inport  Port=4
  HwAg0StepSeqNr : Inport  Port=5
  Abs : Abs
  Add : Sum  Inputs=+-
  CopyRight2 : Subsystem  Description=|  mask(Copyright Information){none=on}
      | Copyright info block.                                               
      |                                                                     
      | Place copyright information at the top of every subsystem in design.
      mask prompts: none "No parameters"
      mask help: Place copyright information at the top of every subsystem in design.
      mask Display:
      | NxtrConf = 'Nexteer Confidential';
      | 
      | sys = bdroot; %handle for the current model ("system")
      | first = get_param(sys,'Created');
      | first = first(end-3:end);  %year is last four digits
      | 
      | last = get_param(sys,'LastModifiedDate');
      | if isempty(last)
      |     last = datestr(now,'yyyy');
      | else
      |     last = last(end-3:end);
      | end
      | 
      | if strcmp(first,last)
      |     fprintf('%s -- Copyright %s Nexteer',NxtrConf,first)
      | else
      |     fprintf('%s -- %s%s- %s Nexteer',NxtrConf,char(169),first,last)
      | end
  Data Store Read1 : DataStoreRead  DataStoreName=HwAg0PrevStepSeqNr
  Data Type Conversion1 : DataTypeConversion  OutDataTypeStr=int8
  Data Type Conversion2 : DataTypeConversion  OutDataTypeStr=int8
  Display : Display
  If : If  IfExpression=(u1 <= 1)|(u1==21)
  "If Action " : Subsystem  TreatAsAtomicUnit=on
  If Action Skip : Subsystem  RequirementInfo={'linktype_rmi_doors' '0000cf45 (/ESG Group/FDD Module Requirements/EA4 Specific/CM690A_HwAg0Meas)' '#CM690A_75' 'true' 'REQ: CM690A_75' '' } %GIDa_9f1636de_fb52_46b4_85d7_aa6c71f2aacb  TreatAsAtomicUnit=on
  Merge : Merge
  Merge1 : Merge
  Merge2 : Merge
  Mux : Mux  Inputs=2
  HwAg0 : Outport  OutDataTypeStr=single
  TestOk : Outport  Port=2  OutDataTypeStr=uint8
  ParamByte : Outport  Port=3  OutDataTypeStr=uint8
  wires:
  HwAg0StepSeqNr/1 -> "If Action "/5(HwAg0StepSeqNr), Mux/1, Data Type Conversion2/1
  Add/1 -> Abs/1
  Abs/1 -> If/1
  If/1 -> "If Action "/Action
  If/2 -> If Action Skip/Action
  Merge/1 -> TestOk/1
  Merge2/1 -> ParamByte/1
  Merge1/1 -> HwAg0/1
  "If Action "/1(HwAg0Meas) -> Merge1/1
  If Action Skip/1(HwAg0Meas) -> Merge1/2
  "If Action "/2(HwAg0TestOk) -> Merge/1
  If Action Skip/2(HwAg0TestOk) -> Merge/2
  "If Action "/3(ParamByte) -> Merge2/1
  If Action Skip/3(ParamByte) -> Merge2/2
  Data Store Read1/1 -> Mux/2, Data Type Conversion1/1
  HwAg0Snsr0Rev/1 -> "If Action "/1(HwAg0Snsr0Rev)
  HwAg0Snsr1Rev/1 -> "If Action "/2(HwAg0Snsr1Rev)
  HwAg0Snsr0Rel/1 -> "If Action "/3(HwAg0Snsr0Rel)
  HwAg0Snsr1Rel/1 -> "If Action "/4(HwAg0Snsr1Rel)
  Mux/1 -> Display/1
  Data Type Conversion1/1 -> Add/2
  Data Type Conversion2/1 -> Add/1

== system CM690A_HwAg0Meas/HwAg0Meas/HwAg0MeasPer4/HwAgRead/If Action Subsystem/AdjStepCalc/InitStep ==
  HwAg0StepSeqNr_In : Inport
  CopyRight2 : Subsystem  Description=|  mask(Copyright Information){none=on}
      | Copyright info block.                                               
      |                                                                     
      | Place copyright information at the top of every subsystem in design.
      mask prompts: none "No parameters"
      mask help: Place copyright information at the top of every subsystem in design.
      mask Display:
      | NxtrConf = 'Nexteer Confidential';
      | 
      | sys = bdroot; %handle for the current model ("system")
      | first = get_param(sys,'Created');
      | first = first(end-3:end);  %year is last four digits
      | 
      | last = get_param(sys,'LastModifiedDate');
      | if isempty(last)
      |     last = datestr(now,'yyyy');
      | else
      |     last = last(end-3:end);
      | end
      | 
      | if strcmp(first,last)
      |     fprintf('%s -- Copyright %s Nexteer',NxtrConf,first)
      | else
      |     fprintf('%s -- %s%s- %s Nexteer',NxtrConf,char(169),first,last)
      | end
  Data Store Read1 : DataStoreRead  DataStoreName=HwAg0InitStepSeqNrCmpl
  DoNothing : Subsystem  TreatAsAtomicUnit=on
  Else : Subsystem  TreatAsAtomicUnit=on
  If : If  IfExpression=u1 == 0
  HwAg0StepSeqNr_Out : Outport
  wires:
  HwAg0StepSeqNr_In/1 -> HwAg0StepSeqNr_Out/1, Else/1(HwAg0StepSeqNr)
  Data Store Read1/1 -> If/1
  If/2 -> DoNothing/Action
  If/1 -> Else/Action

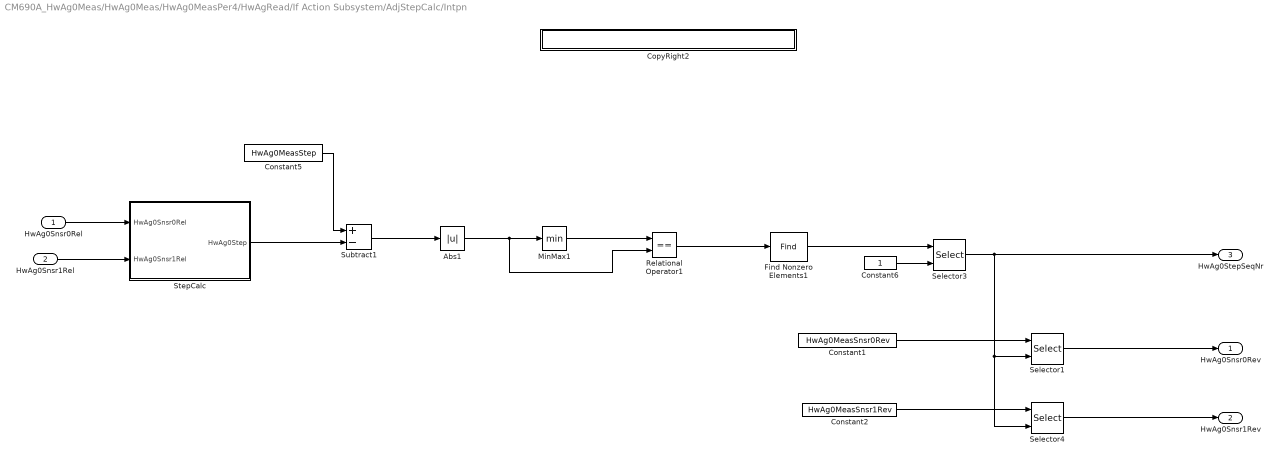
== system CM690A_HwAg0Meas/HwAg0Meas/HwAg0MeasPer4/HwAgRead/If Action Subsystem/AdjStepCalc/Intpn ==
  HwAg0Snsr0Rel : Inport
  HwAg0Snsr1Rel : Inport  Port=2
  Abs1 : Abs
  Constant1 : Constant  Value=HwAg0MeasSnsr0Rev  OutDataTypeStr=int16
  Constant2 : Constant  Value=HwAg0MeasSnsr1Rev  OutDataTypeStr=int16
  Constant5 : Constant  Value=HwAg0MeasStep  OutDataTypeStr=int16
  Constant6 : Constant
  CopyRight2 : Subsystem  Description=|  mask(Copyright Information){none=on}
      | Copyright info block.                                               
      |                                                                     
      | Place copyright information at the top of every subsystem in design.
      mask prompts: none "No parameters"
      mask help: Place copyright information at the top of every subsystem in design.
      mask Display:
      | NxtrConf = 'Nexteer Confidential';
      | 
      | sys = bdroot; %handle for the current model ("system")
      | first = get_param(sys,'Created');
      | first = first(end-3:end);  %year is last four digits
      | 
      | last = get_param(sys,'LastModifiedDate');
      | if isempty(last)
      |     last = datestr(now,'yyyy');
      | else
      |     last = last(end-3:end);
      | end
      | 
      | if strcmp(first,last)
      |     fprintf('%s -- Copyright %s Nexteer',NxtrConf,first)
      | else
      |     fprintf('%s -- %s%s- %s Nexteer',NxtrConf,char(169),first,last)
      | end
  Find Nonzero Elements1 : Find  NumberOfInputDimensions=4  OutDataTypeStr=uint8
  MinMax1 : MinMax
  Relational Operator1 : RelationalOperator  Operator===  OutDataTypeStr=boolean
  Selector1 : Selector  InputPortWidth=22  IndexOptions=Index vector (port)  Indices=[1 3]  OutputSizes=1
  Selector3 : Selector  InputPortWidth=22  IndexOptions=Index vector (port)  Indices=[1 3]  OutputSizes=1
  Selector4 : Selector  InputPortWidth=22  IndexOptions=Index vector (port)  Indices=[1 3]  OutputSizes=1
  StepCalc : Subsystem
  Subtract1 : Sum  Inputs=+-
  HwAg0Snsr0Rev : Outport
  HwAg0Snsr1Rev : Outport  Port=2
  HwAg0StepSeqNr : Outport  Port=3
  wires:
  Subtract1/1 -> Abs1/1
  Constant5/1 -> Subtract1/1
  Abs1/1 -> Relational Operator1/2, MinMax1/1
  Find Nonzero Elements1/1 -> Selector3/1
  Relational Operator1/1 -> Find Nonzero Elements1/1
  MinMax1/1 -> Relational Operator1/1
  Constant6/1 -> Selector3/2
  Constant1/1 -> Selector1/1
  Constant2/1 -> Selector4/1
  Selector1/1 -> HwAg0Snsr0Rev/1
  Selector4/1 -> HwAg0Snsr1Rev/1
  Selector3/1 -> Selector4/2, Selector1/2, HwAg0StepSeqNr/1
  StepCalc/1(HwAg0Step) -> Subtract1/2
  HwAg0Snsr0Rel/1 -> StepCalc/1(HwAg0Snsr0Rel)
  HwAg0Snsr1Rel/1 -> StepCalc/2(HwAg0Snsr1Rel)

== system CM690A_HwAg0Meas/HwAg0Meas/HwAg0MeasPer4/HwAgRead/If Action Subsystem/DebStepSelection/CopyRight2 ==

== system CM690A_HwAg0Meas/HwAg0Meas/HwAg0MeasPer4/HwAgRead/If Action Subsystem/HwAg0Snsr0RelCalc/CopyRight2 ==

== system CM690A_HwAg0Meas/HwAg0Meas/HwAg0MeasPer4/HwAgRead/If Action Subsystem/HwAg0Snsr1RelCalc/CopyRight2 ==

== system CM690A_HwAg0Meas/HwAg0Meas/HwAg0MeasPer4/HwAgRead/If Action Subsystem/SetNtcSts/CopyRight2 ==

== system CM690A_HwAg0Meas/HwAg0Meas/HwAg0MeasPer2/Snsr0Read/RawHwAgRead/NewMsg/NoStsFlt/CommFlt ==
  Action Port : ActionPort  ActionType=else
  Add : Sum
  Bus Creator1 : BusCreator  Inputs=3
  Constant : Constant  OutDataTypeStr=uint8
  CopyRight2 : Subsystem  Description=|  mask(Copyright Information){none=on}
      | Copyright info block.                                               
      |                                                                     
      | Place copyright information at the top of every subsystem in design.
      mask prompts: none "No parameters"
      mask help: Place copyright information at the top of every subsystem in design.
      mask Display:
      | NxtrConf = 'Nexteer Confidential';
      | 
      | sys = bdroot; %handle for the current model ("system")
      | first = get_param(sys,'Created');
      | first = first(end-3:end);  %year is last four digits
      | 
      | last = get_param(sys,'LastModifiedDate');
      | if isempty(last)
      |     last = datestr(now,'yyyy');
      | else
      |     last = last(end-3:end);
      | end
      | 
      | if strcmp(first,last)
      |     fprintf('%s -- Copyright %s Nexteer',NxtrConf,first)
      | else
      |     fprintf('%s -- %s%s- %s Nexteer',NxtrConf,char(169),first,last)
      | end
  Data Store Read : DataStoreRead  DataStoreName=HwAg0Snsr0IntSnsrErrCntr
  Data Store Write : DataStoreWrite  DataStoreName=HwAg0Snsr0IntSnsrErrCntr
  Data Type Conversion : DataTypeConversion  OutDataTypeStr=uint8
  Flt : Constant  Value=ELECGLBPRM_SNSRINTFLT_CNT_U08  OutDataTypeStr=uint8
  HwAg : Constant  Value=0  OutDataTypeStr=uint16
  NtcSts : simulink/Sources/Enumerated Constant  OutDataTypeStr=Enum: NtcSts1  Value=NtcSts1.NTCSTS_PREFAILD  SampleTime=inf
  Signal Conversion1 : SignalConversion
  Out2 : Outport
  wires:
  Flt/1 -> Bus Creator1/3  "ParamByte"
  NtcSts/1 -> Data Type Conversion/1
  HwAg/1 -> Bus Creator1/1  "RawHwAg"
  Bus Creator1/1 -> Signal Conversion1/1
  Signal Conversion1/1 -> Out2/1
  Data Type Conversion/1 -> Bus Creator1/2  "TestOk"
  Data Store Read/1 -> Add/1
  Constant/1 -> Add/2
  Add/1 -> Data Store Write/1

== system CM690A_HwAg0Meas/HwAg0Meas/HwAg0MeasPer2/Snsr0Read/RawHwAgRead/NewMsg/NoStsFlt/CopyRight2 ==
